simulink model "assignment_2"  (R2020b)
settings: Solver=VariableStepAuto  StartTime=1  StopTime=100  RelTol=1e-3
values from neighbouring files (symbols this model uses):
  b = 300    [value.m]
  k1 = 5700    [value.m]
  k2 = 135000    [value.m]
  M1 = 500    [value.m]
  M2 = 50    [value.m]
settings Model: Creator=Sudhanshu  LastModifiedBy=Sudhanshu
settings SolverCC: SolverResetMethod=Robust

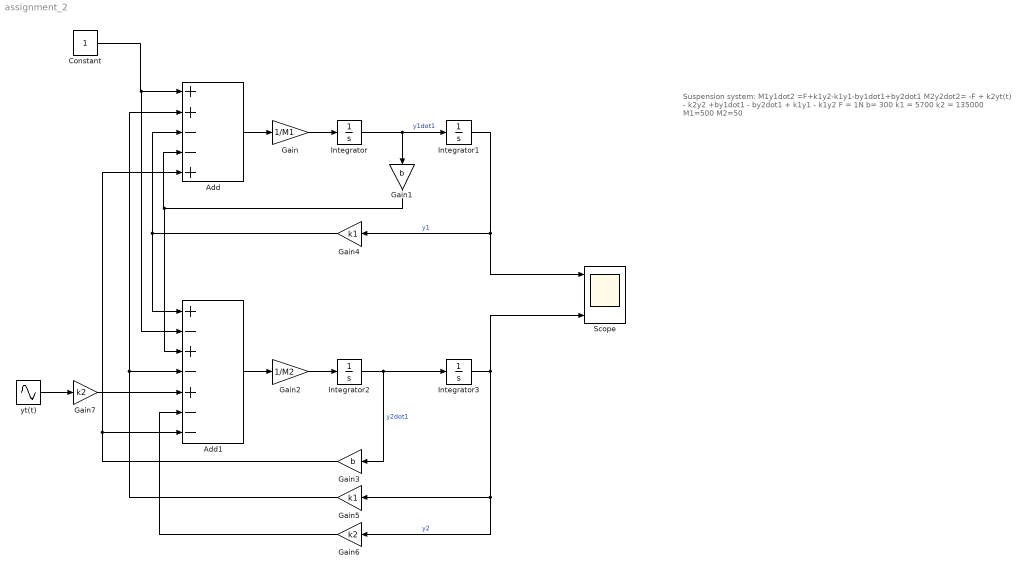
== system assignment_2 ==
  note: Suspension system:
      |
      | M1y1dot2 =F+k1y2-k1y1-by1dot1+by2dot1
      |
      | M2y2dot2= -F + k2yt(t) - k2y2 +by1dot1 - by2dot1 + k1y1 - k1y2
      |
      | F = 1N
      | b= 300
      | k1 = 5700
      | k2 = 135000
      | M1=500
      | M2=50
  Add : Sum  Inputs=++--+
  Add1 : Sum  Inputs=+-+-+--
  Constant : Constant
  Gain : Gain  Gain=1/M1
  Gain1 : Gain  Gain=b
  Gain2 : Gain  Gain=1/M2
  Gain3 : Gain  Gain=b
  Gain4 : Gain  Gain=k1
  Gain5 : Gain  Gain=k1
  Gain6 : Gain  Gain=k2
  Gain7 : Gain  Gain=k2
  Integrator{,1..3} (4 alike) : Integrator
  Scope : Scope  NumInputPorts=3
  yt(t) : Sin  Amplitude=2  Frequency=10  SampleTime=0
  wires:
  Constant/1 -> Add1/2, Add/1
  Add/1 -> Gain/1
  Gain/1 -> Integrator/1
  Integrator/1 -> Gain1/1, Integrator1/1  "y1dot1"
  Gain1/1 -> Add1/3, Add/4
  Add1/1 -> Gain2/1
  Gain2/1 -> Integrator2/1
  Integrator2/1 -> Gain3/1, Integrator3/1  "y2dot1"
  Gain3/1 -> Add/5, Add1/7
  Integrator1/1 -> Scope/1, Gain4/1  "y1"
  Gain4/1 -> Add/3, Add1/1
  Integrator3/1 -> Scope/3, Gain6/1, Gain5/1  "y2"
  Gain5/1 -> Add/2, Add1/4
  Gain6/1 -> Add1/6
  yt(t)/1 -> Gain7/1
  Gain7/1 -> Add1/5
